simulink model "power_battery_aging_sim_SKArizona"  (R2021b)
settings: Solver=ode23tb  StartTime=0.0  StopTime=14400*250  RelTol=1e-3  EnableMultiTasking=on
undefined symbols (not defined in the file or in its folder): Ion, Lithium
libraries: spsStairGeneratorLib x2, spsBatteryLib x1, spsControlledCurrentSourceLib x1, spspowerguiLib x1
settings Model: Creator=The MathWorks, Inc.  LastModifiedBy=CP Gaming1
settings SolverCC: AlgebraicLoopSolver=TrustRegion
settings DataIOCC: LimitDataPoints=on  ReturnWorkspaceOutputs=off
settings OptimizationCC: LifeSpan=inf
settings DebuggingCC: AllowSymbolicDim=off  SFUnexpectedBacktrackingDiag=warning  SFNoUnconditionalDefaultTransitionDiag=warning  SFExecutionAtInitializationDiag=none  SFMachineParentedDataDiag=warning  ArithmeticOperatorsInVariantConditions=warning
settings HardwareCC: ProdBitPerPointer=32  ProdBitPerSizeT=32  ProdBitPerPtrDiffT=32  ProdLargestAtomicFloat=None  ProdIntDivRoundTo=Undefined  ProdEndianess=Unspecified  ProdWordSize=32  ProdHWDeviceType=32-bit Generic
settings ModelReferenceCC: PropagateSignalLabelsOutOfModel=off
settings SFSimCC: SimUseLocalCustomCode=off  CustomCodeUndefinedFunction=UseInterfaceOnly
settings RTWCC: RTWUseLocalCustomCode=off
settings CodeAppCC: StateflowObjectComments=on
settings GRTTargetCC: TargetLangStandard=C89/C90 (ANSI)
settings ConfigComp: CovMetricSettings=dw  CovSaveCumulativeToWorkspaceVar=on  CovSaveSingleToWorkspaceVar=on  CovExternalEMLEnable=off
settings SimscapeCC: SimscapeNormalizeSystem=off

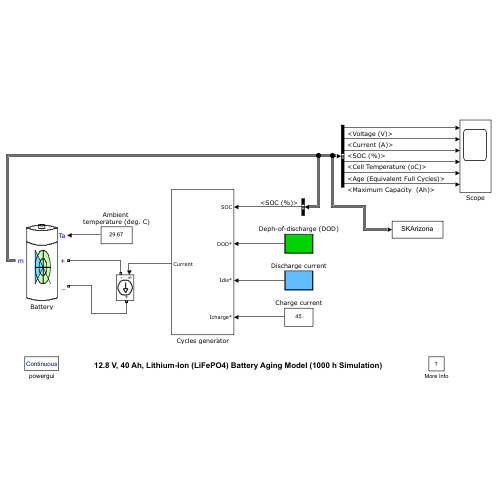
[thumbnail: Simulink's stored preview of the top-level diagram]
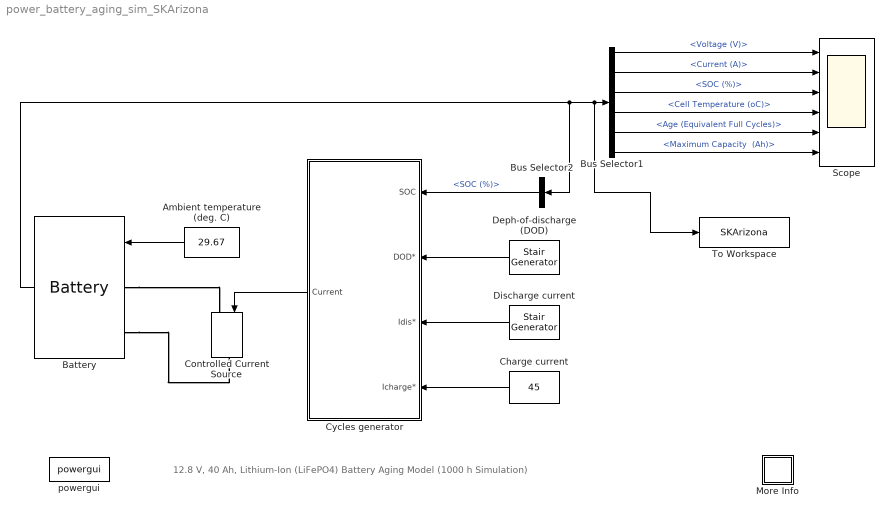
== system power_battery_aging_sim_SKArizona ==
  note: 12.8 V, 40 Ah, Lithium-Ion (LiFePO4) Battery Aging Model (1000 h Simulation)
  Ambient temperature (deg. C) : Constant  Value=29.67
  Battery : spsBatteryLib/Battery  BatType=Lithium-Ion  ShowTempParam=on  ThermalPreset=no  ShowAgeParam=on  NomV=3.7  NomQ=45  SOC=100  Batt_Tr=90  PresetModel=off  MaxQ=45  MinV=2.5  FullV=4.2  Dis_rate=90  R=0.008  Normal_OP=39.76  expZone="[3.94          0.54]"  current=[0.15 1.3 3.25]  Units=Ampere-hour  Tci=25  NomT=20  T2=0  MaxQ2=45  FullV2=4.15  Normal_OP2=3.78  expZone2="[3.94            4]"  Rca=0.178  ti=4880  Dp=0  Neq0=0  Tsim=30  Ta1=23  Qeol=45*0.9  Reol=0.0126*1.2  Char_age=[45, 45.5]  Dis_age=[90, 135]  N1=1500  N2=10445  N3=1017  N4=1460  Ta2=45  N5=982
  Bus Selector1 : BusSelector  OutputSignals="Voltage (V),Current (A),SOC (%),Cell Temperature (oC),Age (Equivalent Full Cycles),Maximum Capacity  (Ah)"
  Bus Selector2 : BusSelector  OutputSignals=SOC (%)
  Charge current : Constant  Value=45
  Controlled Current Source : spsControlledCurrentSourceLib/Controlled Current Source  Initialize=on  Source_Type=AC  Amplitude=0  Phase=0  Frequency=0  Measurements=None
  Cycles generator : Subsystem
  Deph-of-discharge (DOD) : spsStairGeneratorLib/Stair Generator  t=[0 50 100]*14400  e=[20 80 20]  Ts=0
  Discharge current : spsStairGeneratorLib/Stair Generator  t=[0 150 200]*14400  e=[1 4 1]*20  Ts=0
  More Info : Subsystem
      settings: OpenFcn=showdemo(bdroot(gcb))
      mask Display: disp('?')
  Scope : Scope  NumInputPorts=6
  To Workspace : ToWorkspace  VariableName=SKArizona  SaveFormat=Timeseries  SampleTime=-1
  powergui : spspowerguiLib/powergui  SimulationMode=Continuous  SampleTime=0.001  frequency=60  Iterations=50  frequencyindice=0  Pbase=100e6  ErrMax=1e-4  UnitsV=kV  UnitsW=MW  buscounter=0  FunctionMessages=off  echomessages=off  EnableUseOfTLC=off  CurrentSourceSwitches=on  DisableSnubberDevices=off  DisableRonSwitches=off  DisableVfSwitches=off  DisplayEquations=off  AutomaticDiscreteSolvers=off  SolverType=Tustin  Interpol=off  ExternalGateDelay=off  methode=off  Ts=0  x0status=blocks  SPID=off  SwTol=0  HookPort=off  NonlinearTolerance=1e-4  nMaxIteration=100  ContinueOnMaxIteration=off  RestoreLinks=warning  ResistiveCurrentMeasurement=off  Frange=[0:2:500]  Ylog=off  Xlog=on  ShowGrid=off  save=off  variable=ZData  structure=0  ZoomFFT=on  StartTime=0.0  cycles=1  DisplayStyle=1  fundamental=60  FreqAxis=off  MaxFrequency=1000  frequencyindicesteady=1  RmsSteady=1  display=off
  wires:
  Battery/1 -> Bus Selector2/1, To Workspace/1, Bus Selector1/1
  Bus Selector1/1 -> Scope/1  "<Voltage (V)>"
  Bus Selector1/2 -> Scope/2  "<Current (A)>"
  Bus Selector1/3 -> Scope/3  "<SOC (%)>"
  Bus Selector1/4 -> Scope/4  "<Cell Temperature (oC)>"
  Bus Selector1/5 -> Scope/5  "<Age (Equivalent Full Cycles)>"
  Bus Selector1/6 -> Scope/6  "<Maximum Capacity  (Ah)>"
  Cycles generator/1(Current) -> Controlled Current Source/1
  Bus Selector2/1 -> Cycles generator/1(SOC)  "<SOC (%)>"
  Charge current/1 -> Cycles generator/4(Icharge*)
  Deph-of-discharge (DOD)/1 -> Cycles generator/2(DOD*)
  Discharge current/1 -> Cycles generator/3(Idis*)
  Ambient temperature (deg. C)/1 -> Battery/1
  connections:
  Battery/LConn1 -- Controlled Current Source/LConn1
  Battery/LConn2 -- Controlled Current Source/RConn1

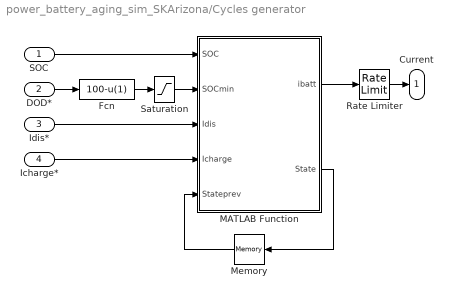
== system power_battery_aging_sim_SKArizona/Cycles generator ==
  SOC : Inport
  DOD* : Inport  Port=2
  Idis* : Inport  Port=3
  Icharge* : Inport  Port=4
  Fcn : Fcn  Expr=100-u(1)
  MATLAB Function : MATLAB Function  TreatAsAtomicUnit=on
  Memory : Memory  InitialCondition=1
  Rate Limiter : RateLimiter  RisingSlewLimit=1000  FallingSlewLimit=-1000  SampleTimeMode=inherited
  Saturation : Saturate  UpperLimit=98  LowerLimit=1
  Current : Outport  VectorParamsAs1DForOutWhenUnconnected=off
  wires:
  MATLAB Function/1(ibatt) -> Rate Limiter/1
  SOC/1 -> MATLAB Function/1(SOC)
  Memory/1 -> MATLAB Function/5(Stateprev)
  MATLAB Function/2(State) -> Memory/1
  DOD*/1 -> Fcn/1
  Fcn/1 -> Saturation/1
  Saturation/1 -> MATLAB Function/2(SOCmin)
  Idis*/1 -> MATLAB Function/3(Idis)
  Icharge*/1 -> MATLAB Function/4(Icharge)
  Rate Limiter/1 -> Current/1

== system power_battery_aging_sim_SKArizona/More Info ==

== matlab function power_battery_aging_sim_SKArizona/Cycles generator/MATLAB Function ==
  data: SOC input; SOCmin input; Idis input; Icharge input; ibatt output; Stateprev input; State output
function [ibatt,State] = fcn(SOC,SOCmin,Idis,Icharge,Stateprev)
%#codegen
State=Stateprev;
if(Stateprev==1 && SOC<=SOCmin)
    State=0;
end
if(Stateprev==0 && SOC>=99)
    State=1;
end
if (Stateprev==1)
    ibatt=Idis;
else
    ibatt=-Icharge;
end
